simulink library "POWER_FACTOR"  (R2024a)
settings: Solver=VariableStepAuto  StartTime=0.0  StopTime=10.0  RelTol=1e-3
settings Model: Creator=gshma  LastModifiedBy=gshma

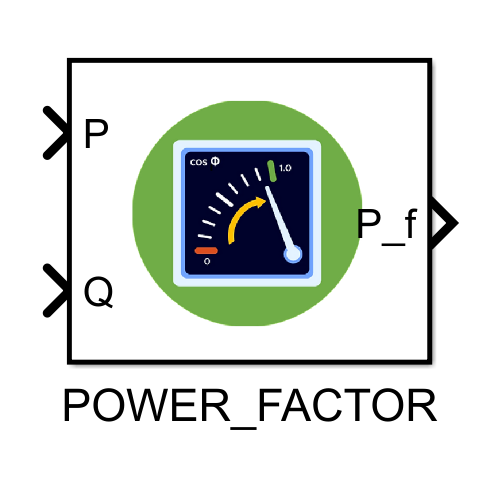
[thumbnail: Simulink's stored preview of the top-level diagram]
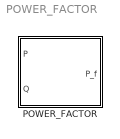
== system POWER_FACTOR ==
  POWER_FACTOR : MATLAB Function  TreatAsAtomicUnit=on

== matlab function POWER_FACTOR/POWER_FACTOR ==
  data: P input; P_f output; Q input
function P_f = POWERFACTOR(P,Q)
    P_f = P/sqrt(P^2+Q^2);
end
